simulink model "SSN_39busRT_Ctrl_4WT_19B"  (R2021a)
settings: Solver=ode3  StartTime=0.0  StopTime=10  FixedStep=Ts  MaxStep=1/60  RelTol=1e-2  AbsTol=1e-1
PreLoadFcn:
  | Ts=2.50e-6; ssn_ieee39_params; load('Pwf.mat');
InitFcn:
  | Ts=2.50e-6; ssn_ieee39_params; load('Pwf.mat');
values from neighbouring files (symbols this model uses):
  f = 50    [ssn_ieee39_params_ctrl.m]
  fNom = f    (= 60)    [ssn_ieee39_params_ctrl.m]
  ILR = 5.02    [ssn_ieee39_params_ctrl.m]
  IQMIN = 0.1    [ssn_ieee39_params_ctrl.m]
  ISCLIM = 1    [ssn_ieee39_params_ctrl.m]
  ITFpu = 1.10    (= 1.1)    [ssn_ieee39_params_ctrl.m]
  K = 1    [ssn_ieee39_params_ctrl.m]
  K1 = 1    [ssn_ieee39_params_ctrl.m]
  K2 = 2    [ssn_ieee39_params_ctrl.m]
  KCL = 1.04    [ssn_ieee39_params_ctrl.m]
  KFB = 0    [ssn_ieee39_params_ctrl.m]
  KFF = 1    [ssn_ieee39_params_ctrl.m]
  KFIX = 1    [ssn_ieee39_params_ctrl.m]
  KG = 1    [ssn_ieee39_params_ctrl.m]
  KIA = 59.91    [ssn_ieee39_params_ctrl.m]
  KIOEX = 0.0303    [ssn_ieee39_params_ctrl.m]
  KIUEX = 0.0303    [ssn_ieee39_params_ctrl.m]
  KIUOEX = 1    [ssn_ieee39_params_ctrl.m]
  KIUUEX = 1    [ssn_ieee39_params_ctrl.m]
  KLR = 22.47    [ssn_ieee39_params_ctrl.m]
  KM = 1    [ssn_ieee39_params_ctrl.m]
  KOEL = 0.24    [ssn_ieee39_params_ctrl.m]
  Kp = 1    [ssn_ieee39_params_ctrl.m]
  KPA = 30    [ssn_ieee39_params_ctrl.m]
  KPOEL = 1    [ssn_ieee39_params_ctrl.m]
  KPOEX = 0    [ssn_ieee39_params_ctrl.m]
  KPUEX = 0    [ssn_ieee39_params_ctrl.m]
  KSCALE = 0.319    [ssn_ieee39_params_ctrl.m]
  KUF = 0    [ssn_ieee39_params_ctrl.m]
  KUI = 0.001    [ssn_ieee39_params_ctrl.m]
  KUL = 0.24    [ssn_ieee39_params_ctrl.m]
  s = 10    [ssn_ieee39_params_ctrl.m]
  TA = 0.01    [ssn_ieee39_params_ctrl.m]
  Tadj = 0    [ssn_ieee39_params_ctrl.m]
  taps = [1 1 1.07 1.07 1.009 1.025 1 1.025 1.025 1.025]*1    [ssn_ieee39_params_ctrl.m]
  TF = 0.02    [ssn_ieee39_params_ctrl.m]
  TG = 0.024    [ssn_ieee39_params_ctrl.m]
  TINV = 0    [ssn_ieee39_params_ctrl.m]
  TIT = 0.1    [ssn_ieee39_params_ctrl.m]
  TL_10_11_len = 14    [ssn_ieee39_params_ctrl.m]
  TL_10_13_len = 14    [ssn_ieee39_params_ctrl.m]
  TL_13_14_len = 32    [ssn_ieee39_params_ctrl.m]
  TL_14_15_len = 70    [ssn_ieee39_params_ctrl.m]
  TL_15_16_len = 31.5    [ssn_ieee39_params_ctrl.m]
  TL_16_17_len = 26    [ssn_ieee39_params_ctrl.m]
  TL_16_19_len = 61    [ssn_ieee39_params_ctrl.m]
  TL_16_21_len = 46    [ssn_ieee39_params_ctrl.m]
  TL_16_24_len = 15    [ssn_ieee39_params_ctrl.m]
  TL_17_18_len = 26    [ssn_ieee39_params_ctrl.m]
  TL_17_27_len = 59    [ssn_ieee39_params_ctrl.m]
  TL_1_2_len = 134    [ssn_ieee39_params_ctrl.m]
  TL_1_39_len = 105    [ssn_ieee39_params_ctrl.m]
  TL_21_22_len = 47    [ssn_ieee39_params_ctrl.m]
  TL_22_23_len = 33    [ssn_ieee39_params_ctrl.m]
  TL_24_23_len = 88    [ssn_ieee39_params_ctrl.m]
  TL_25_26_len = 101    [ssn_ieee39_params_ctrl.m]
  TL_26_27_len = 46.5    [ssn_ieee39_params_ctrl.m]
  TL_26_28_len = 151    [ssn_ieee39_params_ctrl.m]
  TL_26_29_len = 200    [ssn_ieee39_params_ctrl.m]
  TL_28_29_len = 48    [ssn_ieee39_params_ctrl.m]
  TL_2_25_len = 28    [ssn_ieee39_params_ctrl.m]
  TL_2_2_len = 49    [ssn_ieee39_params_ctrl.m]
  TL_3_18_len = 42    [ssn_ieee39_params_ctrl.m]
  TL_3_4_len = 53    [ssn_ieee39_params_ctrl.m]
  TL_4_14_len = 33    [ssn_ieee39_params_ctrl.m]
  TL_4_5_len = 32.5    [ssn_ieee39_params_ctrl.m]
  TL_5_6_len = 14    [ssn_ieee39_params_ctrl.m]
  TL_5_8_len = 32    [ssn_ieee39_params_ctrl.m]
  TL_6_11_len = 26.5    [ssn_ieee39_params_ctrl.m]
  TL_6_7_len = 25.5    [ssn_ieee39_params_ctrl.m]
  TL_7_8_len = 15    [ssn_ieee39_params_ctrl.m]
  TL_8_9_len = 93    [ssn_ieee39_params_ctrl.m]
  TL_9_39_len = 136    [ssn_ieee39_params_ctrl.m]
  TOEL = 5.00    (= 5)    [ssn_ieee39_params_ctrl.m]
  TQREF = 0    [ssn_ieee39_params_ctrl.m]
  TQSCL = 0.012    [ssn_ieee39_params_ctrl.m]
  Ts_PMU = 1/1000    (= 0.001)    [ssn_ieee39_params_ctrl.m]
  TU1 = 0    [ssn_ieee39_params_ctrl.m]
  TU2 = 0    [ssn_ieee39_params_ctrl.m]
  TU3 = 0    [ssn_ieee39_params_ctrl.m]
  TU4 = 0    [ssn_ieee39_params_ctrl.m]
  TUL = 0    [ssn_ieee39_params_ctrl.m]
  TUP = 0.050    (= 0.05)    [ssn_ieee39_params_ctrl.m]
  TUQ = .005    (= 0.005)    [ssn_ieee39_params_ctrl.m]
  TUV = 0.2    [ssn_ieee39_params_ctrl.m]
  VAAMAX = VAMAX    (= 7.05)    [ssn_ieee39_params_ctrl.m]
  VAMAX = 7.05    [ssn_ieee39_params_ctrl.m]
  VAMIN = -6.11    [ssn_ieee39_params_ctrl.m]
  VBMAX = 999    [ssn_ieee39_params_ctrl.m]
  VF = 0    [ssn_ieee39_params_ctrl.m]
  VFB = 0    [ssn_ieee39_params_ctrl.m]
  VMMAX = 7.05    [ssn_ieee39_params_ctrl.m]
  VMMIN = -6.11    [ssn_ieee39_params_ctrl.m]
  VOELmax1 = 0.2353    [ssn_ieee39_params_ctrl.m]
  VOELmax2 = 0.0    (= 0)    [ssn_ieee39_params_ctrl.m]
  VOELmin1 = -0.24    [ssn_ieee39_params_ctrl.m]
  VOELmin2 = -1.0    (= -1)    [ssn_ieee39_params_ctrl.m]
  VRMAX = 7.05    [ssn_ieee39_params_ctrl.m]
  VRMIN = -6.11    [ssn_ieee39_params_ctrl.m]
  VSCLmax = 0.20    (= 0.2)    [ssn_ieee39_params_ctrl.m]
  VSCLmin = -0.10    (= -0.1)    [ssn_ieee39_params_ctrl.m]
  VUELmax1 = 1    [ssn_ieee39_params_ctrl.m]
  VUELmax2 = 1    [ssn_ieee39_params_ctrl.m]
  VUELmin1 = -1    [ssn_ieee39_params_ctrl.m]
  VUELmin2 = -1    [ssn_ieee39_params_ctrl.m]
  VUImax = 1    [ssn_ieee39_params_ctrl.m]
  VUImin = -1    [ssn_ieee39_params_ctrl.m]
undefined symbols (not defined in the file or in its folder): another_event_name, D1, Delta, DiscIntNeverNeededParam, find_system, MOV_segment9, my_event_name, powergui, Pw1, Pw2, Pw3, Pw4, vNomHV
libraries: powerlib_extras x162, spsThreePhaseVIMeasurementLib x55, spsCurrentMeasurementLib x52, simulink_extras x44, slpidlib x40, op_dpl_lib x36, spsST2AModel x20, spsThreePhaseParallelRLCLoadLib x20, spsThreePhaseTransformerTwoWindingsLib x17, spsControlledVoltageSourceLib x16, spsVoltageMeasurementLib x12, spsSynchronousMachinepuStandardLib x10
(part 15 of 19)

== system SSN_39busRT_Ctrl_4WT_19B/SM_master/4 WT/SS_windfarm3to4/Wind Farm (DFIG Type)/Wind Turbine Doubly-Fed Induction Generator (Average Model)1/Average_VSC ==
  Uref : Inport
  Converter_model : Subsystem
  Demux : Demux  Outputs=2
  Ia_meas : spsCurrentMeasurementLib/Current Measurement  PhasorSimulation=off  OutputType=Complex  PSBequivalent=0
  Ic_meas : spsCurrentMeasurementLib/Current Measurement  PhasorSimulation=off  OutputType=Complex  PSBequivalent=0
  Idc : spsControlledCurrentSourceLib/Controlled Current Source  Initialize=on  Source_Type=AC  Amplitude=0  Phase=0  Frequency=0  Measurements=None
  Mux : Mux  Inputs=2
  Vab : spsControlledVoltageSourceLib/Controlled Voltage Source  Initialize=on  Source_Type=AC  Amplitude=0  Phase=0  Frequency=0  Measurements=None
  Vbc : spsControlledVoltageSourceLib/Controlled Voltage Source  Initialize=on  Source_Type=AC  Amplitude=0  Phase=0  Frequency=0  Measurements=None
  Vdc_meas : spsVoltageMeasurementLib/Voltage Measurement  PhasorSimulation=off  OutputType=Complex  PSBequivalent=0
  A : PMIOPort  Side=Left
  B : PMIOPort  Port=2  Side=Left
  C : PMIOPort  Port=3  Side=Left
  + : PMIOPort  Port=4  Side=Right
  - : PMIOPort  Port=5  Side=Right
  wires:
  Converter_model/2(Vab_Vbc) -> Demux/1
  Converter_model/1(Idc) -> Idc/1  "Idc"
  Mux/1 -> Converter_model/1(Ia_Ic)
  Vdc_meas/1 -> Converter_model/2(Vdc)
  Uref/1 -> Converter_model/3(Uref)
  Ic_meas/1 -> Mux/2  "Ic"
  Ia_meas/1 -> Mux/1  "Ia"
  Demux/1 -> Vab/1  "Vab"
  Demux/2 -> Vbc/1  "Vbc"
  connections:
  Idc/LConn1 -- -/RConn1 -- Vdc_meas/LConn1
  Idc/RConn1 -- +/RConn1 -- Vdc_meas/LConn2
  C/RConn1 -- Ic_meas/LConn1
  A/RConn1 -- Ia_meas/LConn1
  Ia_meas/RConn1 -- Vab/LConn1
  B/RConn1 -- Vbc/LConn1 -- Vab/RConn1
  Vbc/RConn1 -- Ic_meas/RConn1

== system SSN_39busRT_Ctrl_4WT_19B/SM_master/4 WT/SS_windfarm3to4/Wind Farm (DFIG Type)/Wind Turbine Doubly-Fed Induction Generator (Average Model)1/Average_VSC1 ==
  Uref : Inport
  Converter_model : Subsystem
  Demux : Demux  Outputs=2
  Ia_meas : spsCurrentMeasurementLib/Current Measurement  PhasorSimulation=off  OutputType=Complex  PSBequivalent=0
  Ic_meas : spsCurrentMeasurementLib/Current Measurement  PhasorSimulation=off  OutputType=Complex  PSBequivalent=0
  Idc : spsControlledCurrentSourceLib/Controlled Current Source  Initialize=on  Source_Type=AC  Amplitude=0  Phase=0  Frequency=0  Measurements=None
  Mux : Mux  Inputs=2
  Vab : spsControlledVoltageSourceLib/Controlled Voltage Source  Initialize=on  Source_Type=AC  Amplitude=0  Phase=0  Frequency=0  Measurements=None
  Vbc : spsControlledVoltageSourceLib/Controlled Voltage Source  Initialize=on  Source_Type=AC  Amplitude=0  Phase=0  Frequency=0  Measurements=None
  Vdc_meas : spsVoltageMeasurementLib/Voltage Measurement  PhasorSimulation=off  OutputType=Complex  PSBequivalent=0
  A : PMIOPort  Side=Left
  B : PMIOPort  Port=2  Side=Left
  C : PMIOPort  Port=3  Side=Left
  + : PMIOPort  Port=4  Side=Right
  - : PMIOPort  Port=5  Side=Right
  wires:
  Converter_model/2(Vab_Vbc) -> Demux/1
  Converter_model/1(Idc) -> Idc/1  "Idc"
  Mux/1 -> Converter_model/1(Ia_Ic)
  Vdc_meas/1 -> Converter_model/2(Vdc)
  Uref/1 -> Converter_model/3(Uref)
  Ic_meas/1 -> Mux/2  "Ic"
  Ia_meas/1 -> Mux/1  "Ia"
  Demux/1 -> Vab/1  "Vab"
  Demux/2 -> Vbc/1  "Vbc"
  connections:
  Idc/LConn1 -- -/RConn1 -- Vdc_meas/LConn1
  Idc/RConn1 -- +/RConn1 -- Vdc_meas/LConn2
  C/RConn1 -- Ic_meas/LConn1
  A/RConn1 -- Ia_meas/LConn1
  Ia_meas/RConn1 -- Vab/LConn1
  B/RConn1 -- Vbc/LConn1 -- Vab/RConn1
  Vbc/RConn1 -- Ic_meas/RConn1

== system SSN_39busRT_Ctrl_4WT_19B/SM_master/4 WT/SS_windfarm3to4/Wind Farm (DFIG Type)/Wind Turbine Doubly-Fed Induction Generator (Average Model)1/Control System_average ==
  Vabc_B1 : Inport
  Q_ref : Inport  Port=2
  Iq_grid_conv_ref : Inport  Port=3
  wr : Inport  Port=4
  Iabc_grid_conv : Inport  Port=5
  Iabc_stator : Inport  Port=6
  Iabc_rotor : Inport  Port=7
  Q_B1 : Inport  Port=8
  angle_rotor : Inport  Port=9
  Vdc : Inport  Port=10
  Control : Subsystem
  Filter 1000 Hz : Subsystem  mask{Freq=1000, Zeta=0.707, Ts=Ts}
      mask prompts: Freq "Cut-off frequency (Hz):"; Zeta "Damping factor Zeta:"; Ts "Sample time"
  Unit Delay3 : UnitDelay  SampleTime=Ts  HasFrameUpgradeWarning=on
  Unit Delay4 : UnitDelay  SampleTime=Ts  HasFrameUpgradeWarning=on
  Uref_grid_conv : Outport
  Uref_rotor_conv : Outport  Port=2
  Theta_Freq : Outport  Port=3
  Pitch_angle : Outport  Port=4
  wires:
  wr/1 -> Filter 1000 Hz/9(wr)
  Q_B1/1 -> Filter 1000 Hz/8(Q_B1)
  Iabc_grid_conv/1 -> Filter 1000 Hz/2(Iabc_grid_conv)
  Iabc_rotor/1 -> Filter 1000 Hz/5(Iabc_rotor)
  Filter 1000 Hz/1("Vabc_B1 ") -> Control/1(Vabc_B1)
  Filter 1000 Hz/2("Iabc_grid_conv ") -> Control/2(Iabc_grid_conv)
  Filter 1000 Hz/3("Vdc ") -> Control/3(Vdc)
  Filter 1000 Hz/4("Iabc_stator ") -> Control/4(Iabc_stator)
  Filter 1000 Hz/5("Iabc_rotor ") -> Control/5(Iabc_rotor)
  Filter 1000 Hz/6("Q_ref ") -> Control/6(Q_ref)
  Filter 1000 Hz/7("Iq_grid_conv_ref ") -> Control/7(Iq_grid_conv_ref)
  Filter 1000 Hz/8("Q_B1 ") -> Control/8(Q_B1)
  Filter 1000 Hz/9("wr ") -> Control/9(wr)
  Filter 1000 Hz/10("angle_rotor ") -> Control/10(angle_rotor)
  Vabc_B1/1 -> Filter 1000 Hz/1(Vabc_B1)
  Iabc_stator/1 -> Filter 1000 Hz/4(Iabc_stator)
  Q_ref/1 -> Filter 1000 Hz/6(Q_ref)
  Iq_grid_conv_ref/1 -> Filter 1000 Hz/7(Iq_grid_conv_ref)
  Control/3(Theta_Freq) -> Theta_Freq/1
  Control/4(Pitch_angle) -> Pitch_angle/1
  Control/1(Uctrl_grid_conv) -> Unit Delay4/1
  Control/2(Uctrl_rotor_conv) -> Unit Delay3/1
  Vdc/1 -> Filter 1000 Hz/3(Vdc)
  angle_rotor/1 -> Filter 1000 Hz/10(angle_rotor)
  Unit Delay4/1 -> Uref_grid_conv/1
  Unit Delay3/1 -> Uref_rotor_conv/1

== system SSN_39busRT_Ctrl_4WT_19B/SM_master/4 WT/SS_windfarm3to4/Wind Farm (DFIG Type)/Wind Turbine Doubly-Fed Induction Generator (Average Model)1/Data acquisition electrical ==
  Vabc_B1 : Inport
  Iabc_B1 : Inport  Port=2
  Theta_Freq : Inport  Port=3
  Vdc : Inport  Port=4
  -->pu : Gain  Gain=1/(Pnom*NumberOfUnits)  SaturateOnIntegerOverflow=on  OutDataTypeStr=Inherit: Same as input  ParamDataTypeStr=Inherit: Same as input
  -1 : Gain  Gain=-1  SaturateOnIntegerOverflow=on  OutDataTypeStr=Inherit: Same as input  ParamDataTypeStr=Inherit: Same as input
  Bus Creator : BusCreator  Inputs=5
  Demux1 : Demux  Outputs=2
      settings: DisplayOption=none
  Demux2 : Demux  Outputs=2
      settings: DisplayOption=none
  Discrete 3-phase PLL-Driven Positive-Sequence Active & Reactive Power : powerlib_extras/Discrete Measurements/Discrete 3-phase PLL-Driven  Positive-Sequence Active & Reactive Power  Finit=Fnom  Fmin=45  Par_Vinit=[1 30]  Par_Iinit=[0.5 -10]  Ts=Ts_Control
      settings: SourceProductBaseCode=PS
  Mux : Mux  Inputs=2
  Terminator : Terminator
  Trigonometric Function : Trigonometry
  Trigonometric Function1 : Trigonometry  Operator=cos
  pu->A : Gain  Gain=Pnom*NumberOfUnits/sqrt(3)/Vnom*sqrt(2)  SaturateOnIntegerOverflow=on  OutDataTypeStr=Inherit: Same as input  ParamDataTypeStr=Inherit: Same as input
  pu->V : Gain  Gain=Vnom*sqrt(2)/sqrt(3)  SaturateOnIntegerOverflow=on  OutDataTypeStr=Inherit: Same as input  ParamDataTypeStr=Inherit: Same as input
  meas : Outport
  Q_B1 : Outport  Port=2
  wires:
  Demux2/2 -> Discrete 3-phase PLL-Driven Positive-Sequence Active & Reactive Power/1
  Demux2/1 -> Trigonometric Function1/1, Trigonometric Function/1
  Theta_Freq/1 -> Demux2/1
  Discrete 3-phase PLL-Driven Positive-Sequence Active & Reactive Power/1 -> Terminator/1
  Mux/1 -> Discrete 3-phase PLL-Driven Positive-Sequence Active & Reactive Power/2
  Trigonometric Function1/1 -> Mux/2
  Trigonometric Function/1 -> Mux/1
  pu->V/1 -> Discrete 3-phase PLL-Driven Positive-Sequence Active & Reactive Power/3
  Discrete 3-phase PLL-Driven Positive-Sequence Active & Reactive Power/2 -> -1/1
  pu->A/1 -> Discrete 3-phase PLL-Driven Positive-Sequence Active & Reactive Power/4
  Bus Creator/1 -> meas/1
  Iabc_B1/1 -> pu->A/1, Bus Creator/2  "Iabc_B1"
  Vabc_B1/1 -> pu->V/1, Bus Creator/1  "Vabc_B1"
  Vdc/1 -> Bus Creator/5  "Vdc"
  -1/1 -> Demux1/1
  Demux1/2 -> Bus Creator/4, -->pu/1  "Q_B1"
  Demux1/1 -> Bus Creator/3  "P_B1"
  -->pu/1 -> Q_B1/1

== system SSN_39busRT_Ctrl_4WT_19B/SM_master/4 WT/SS_windfarm3to4/Wind Farm (DFIG Type)/Wind Turbine Doubly-Fed Induction Generator (Average Model)1/Subsystem ==
  Current Measurement : spsCurrentMeasurementLib/Current Measurement  PhasorSimulation=off  OutputType=Complex  PSBequivalent=0
  Current Measurement1 : spsCurrentMeasurementLib/Current Measurement  PhasorSimulation=off  OutputType=Complex  PSBequivalent=0
  Current Measurement2 : spsCurrentMeasurementLib/Current Measurement  PhasorSimulation=off  OutputType=Complex  PSBequivalent=0
  Gain : Gain  Gain=1/(Pnom*NumberOfUnits/(Vnom*sqrt(3)))/sqrt(2)
  Mux : Mux  Inputs=3
  A : PMIOPort  Side=Left
  a : PMIOPort  Port=2  Side=Right
  B : PMIOPort  Port=3  Side=Left
  b : PMIOPort  Port=4  Side=Right
  C : PMIOPort  Port=5  Side=Left
  c : PMIOPort  Port=6  Side=Right
  IabcPU : Outport
  wires:
  Current Measurement2/1 -> Mux/3
  Current Measurement1/1 -> Mux/2
  Current Measurement/1 -> Mux/1
  Mux/1 -> Gain/1
  Gain/1 -> IabcPU/1
  connections:
  A/RConn1 -- Current Measurement/LConn1
  a/RConn1 -- Current Measurement/RConn1
  b/RConn1 -- Current Measurement1/RConn1
  B/RConn1 -- Current Measurement1/LConn1
  C/RConn1 -- Current Measurement2/LConn1
  c/RConn1 -- Current Measurement2/RConn1

== system SSN_39busRT_Ctrl_4WT_19B/SM_master/4 WT/SS_windfarm3to4/Wind Farm (DFIG Type)/Wind Turbine Doubly-Fed Induction Generator (Average Model)1/Subsystem1 ==
  Current Measurement : spsCurrentMeasurementLib/Current Measurement  PhasorSimulation=off  OutputType=Complex  PSBequivalent=0
  Current Measurement1 : spsCurrentMeasurementLib/Current Measurement  PhasorSimulation=off  OutputType=Complex  PSBequivalent=0
  Current Measurement2 : spsCurrentMeasurementLib/Current Measurement  PhasorSimulation=off  OutputType=Complex  PSBequivalent=0
  Gain : Gain  Gain=1/(Pnom*NumberOfUnits/(Vnom*sqrt(3)))/sqrt(2)
  Mux : Mux  Inputs=3
  A : PMIOPort  Side=Left
  a : PMIOPort  Port=2  Side=Right
  B : PMIOPort  Port=3  Side=Left
  b : PMIOPort  Port=4  Side=Right
  C : PMIOPort  Port=5  Side=Left
  c : PMIOPort  Port=6  Side=Right
  IabcPU : Outport
  wires:
  Gain/1 -> IabcPU/1
  Mux/1 -> Gain/1
  Current Measurement/1 -> Mux/1
  Current Measurement1/1 -> Mux/2
  Current Measurement2/1 -> Mux/3
  connections:
  c/RConn1 -- Current Measurement2/RConn1
  C/RConn1 -- Current Measurement2/LConn1
  B/RConn1 -- Current Measurement1/LConn1
  b/RConn1 -- Current Measurement1/RConn1
  a/RConn1 -- Current Measurement/RConn1
  A/RConn1 -- Current Measurement/LConn1

== system SSN_39busRT_Ctrl_4WT_19B/SM_master/4 WT/SS_windfarm3to4/Wind Farm (DFIG Type)/Wind Turbine Doubly-Fed Induction Generator (Average Model)1/Subsystem2 ==
  Current Measurement : spsCurrentMeasurementLib/Current Measurement  PhasorSimulation=off  OutputType=Complex  PSBequivalent=0
  Current Measurement1 : spsCurrentMeasurementLib/Current Measurement  PhasorSimulation=off  OutputType=Complex  PSBequivalent=0
  Current Measurement2 : spsCurrentMeasurementLib/Current Measurement  PhasorSimulation=off  OutputType=Complex  PSBequivalent=0
  Gain : Gain  Gain=1/(Pnom*NumberOfUnits/(Vnom*sqrt(3)))/sqrt(2)
  Mux : Mux  Inputs=3
  A : PMIOPort  Side=Left
  a : PMIOPort  Port=2  Side=Right
  B : PMIOPort  Port=3  Side=Left
  b : PMIOPort  Port=4  Side=Right
  C : PMIOPort  Port=5  Side=Left
  c : PMIOPort  Port=6  Side=Right
  IabcPU : Outport
  wires:
  Current Measurement2/1 -> Mux/3
  Current Measurement1/1 -> Mux/2
  Current Measurement/1 -> Mux/1
  Mux/1 -> Gain/1
  Gain/1 -> IabcPU/1
  connections:
  A/RConn1 -- Current Measurement/LConn1
  a/RConn1 -- Current Measurement/RConn1
  b/RConn1 -- Current Measurement1/RConn1
  B/RConn1 -- Current Measurement1/LConn1
  C/RConn1 -- Current Measurement2/LConn1
  c/RConn1 -- Current Measurement2/RConn1

== system SSN_39busRT_Ctrl_4WT_19B/SM_master/4 WT/SS_windfarm3to4/Wind Farm (DFIG Type)/Wind Turbine Doubly-Fed Induction Generator (Average Model)1/Wind Turbine v ==
  Generator speed (pu) : Inport
  Wind Power : Inport  Port=2
  Avoid division by zero : Saturate  UpperLimit=1e6  LowerLimit=1e-6
  Gain : Gain  Gain=-1  SaturateOnIntegerOverflow=on  OutDataTypeStr=Inherit: Same as input  ParamDataTypeStr=Inherit: Same as input
  Product2 : Product  Inputs=*/  InputSameDT=on  SaturateOnIntegerOverflow=on  OutDataTypeStr=Inherit: Same as first input
  pu->pu : Gain  Gain=P_wind_base*Pnom/Pelec_base  SaturateOnIntegerOverflow=on  OutDataTypeStr=Inherit: Same as input  ParamDataTypeStr=Inherit: Same as input
  Tm (pu) : Outport
  wires:
  Generator speed (pu)/1 -> Avoid division by zero/1
  pu->pu/1 -> Product2/1
  Gain/1 -> Tm (pu)/1
  Avoid division by zero/1 -> Product2/2
  Product2/1 -> Gain/1
  Wind Power/1 -> pu->pu/1

== system SSN_39busRT_Ctrl_4WT_19B/SM_master/4 WT/SS_windfarm3to4/Wind Farm (DFIG Type)2/Wind Turbine Doubly-Fed Induction Generator (Average Model)1/Average_VSC ==
  Uref : Inport
  Converter_model : Subsystem
  Demux : Demux  Outputs=2
  Ia_meas : spsCurrentMeasurementLib/Current Measurement  PhasorSimulation=off  OutputType=Complex  PSBequivalent=0
  Ic_meas : spsCurrentMeasurementLib/Current Measurement  PhasorSimulation=off  OutputType=Complex  PSBequivalent=0
  Idc : spsControlledCurrentSourceLib/Controlled Current Source  Initialize=on  Source_Type=AC  Amplitude=0  Phase=0  Frequency=0  Measurements=None
  Mux : Mux  Inputs=2
  Vab : spsControlledVoltageSourceLib/Controlled Voltage Source  Initialize=on  Source_Type=AC  Amplitude=0  Phase=0  Frequency=0  Measurements=None
  Vbc : spsControlledVoltageSourceLib/Controlled Voltage Source  Initialize=on  Source_Type=AC  Amplitude=0  Phase=0  Frequency=0  Measurements=None
  Vdc_meas : spsVoltageMeasurementLib/Voltage Measurement  PhasorSimulation=off  OutputType=Complex  PSBequivalent=0
  A : PMIOPort  Side=Left
  B : PMIOPort  Port=2  Side=Left
  C : PMIOPort  Port=3  Side=Left
  + : PMIOPort  Port=4  Side=Right
  - : PMIOPort  Port=5  Side=Right
  wires:
  Demux/2 -> Vbc/1  "Vbc"
  Demux/1 -> Vab/1  "Vab"
  Ia_meas/1 -> Mux/1  "Ia"
  Ic_meas/1 -> Mux/2  "Ic"
  Uref/1 -> Converter_model/3(Uref)
  Vdc_meas/1 -> Converter_model/2(Vdc)
  Mux/1 -> Converter_model/1(Ia_Ic)
  Converter_model/1(Idc) -> Idc/1  "Idc"
  Converter_model/2(Vab_Vbc) -> Demux/1
  connections:
  Vbc/RConn1 -- Ic_meas/RConn1
  Vab/RConn1 -- Vbc/LConn1 -- B/RConn1
  Ia_meas/RConn1 -- Vab/LConn1
  A/RConn1 -- Ia_meas/LConn1
  C/RConn1 -- Ic_meas/LConn1
  Vdc_meas/LConn2 -- +/RConn1 -- Idc/RConn1
  Vdc_meas/LConn1 -- -/RConn1 -- Idc/LConn1

== system SSN_39busRT_Ctrl_4WT_19B/SM_master/4 WT/SS_windfarm3to4/Wind Farm (DFIG Type)2/Wind Turbine Doubly-Fed Induction Generator (Average Model)1/Average_VSC1 ==
  Uref : Inport
  Converter_model : Subsystem
  Demux : Demux  Outputs=2
  Ia_meas : spsCurrentMeasurementLib/Current Measurement  PhasorSimulation=off  OutputType=Complex  PSBequivalent=0
  Ic_meas : spsCurrentMeasurementLib/Current Measurement  PhasorSimulation=off  OutputType=Complex  PSBequivalent=0
  Idc : spsControlledCurrentSourceLib/Controlled Current Source  Initialize=on  Source_Type=AC  Amplitude=0  Phase=0  Frequency=0  Measurements=None
  Mux : Mux  Inputs=2
  Vab : spsControlledVoltageSourceLib/Controlled Voltage Source  Initialize=on  Source_Type=AC  Amplitude=0  Phase=0  Frequency=0  Measurements=None
  Vbc : spsControlledVoltageSourceLib/Controlled Voltage Source  Initialize=on  Source_Type=AC  Amplitude=0  Phase=0  Frequency=0  Measurements=None
  Vdc_meas : spsVoltageMeasurementLib/Voltage Measurement  PhasorSimulation=off  OutputType=Complex  PSBequivalent=0
  A : PMIOPort  Side=Left
  B : PMIOPort  Port=2  Side=Left
  C : PMIOPort  Port=3  Side=Left
  + : PMIOPort  Port=4  Side=Right
  - : PMIOPort  Port=5  Side=Right
  wires:
  Demux/2 -> Vbc/1  "Vbc"
  Demux/1 -> Vab/1  "Vab"
  Ia_meas/1 -> Mux/1  "Ia"
  Ic_meas/1 -> Mux/2  "Ic"
  Uref/1 -> Converter_model/3(Uref)
  Vdc_meas/1 -> Converter_model/2(Vdc)
  Mux/1 -> Converter_model/1(Ia_Ic)
  Converter_model/1(Idc) -> Idc/1  "Idc"
  Converter_model/2(Vab_Vbc) -> Demux/1
  connections:
  Vbc/RConn1 -- Ic_meas/RConn1
  Vab/RConn1 -- Vbc/LConn1 -- B/RConn1
  Ia_meas/RConn1 -- Vab/LConn1
  A/RConn1 -- Ia_meas/LConn1
  C/RConn1 -- Ic_meas/LConn1
  Vdc_meas/LConn2 -- +/RConn1 -- Idc/RConn1
  Vdc_meas/LConn1 -- -/RConn1 -- Idc/LConn1

== system SSN_39busRT_Ctrl_4WT_19B/SM_master/4 WT/SS_windfarm3to4/Wind Farm (DFIG Type)2/Wind Turbine Doubly-Fed Induction Generator (Average Model)1/Control System_average ==
  Vabc_B1 : Inport
  Q_ref : Inport  Port=2
  Iq_grid_conv_ref : Inport  Port=3
  wr : Inport  Port=4
  Iabc_grid_conv : Inport  Port=5
  Iabc_stator : Inport  Port=6
  Iabc_rotor : Inport  Port=7
  Q_B1 : Inport  Port=8
  angle_rotor : Inport  Port=9
  Vdc : Inport  Port=10
  Control : Subsystem
  Filter 1000 Hz : Subsystem  mask{Freq=1000, Zeta=0.707, Ts=Ts}
      mask prompts: Freq "Cut-off frequency (Hz):"; Zeta "Damping factor Zeta:"; Ts "Sample time"
  Unit Delay3 : UnitDelay  SampleTime=Ts  HasFrameUpgradeWarning=on
  Unit Delay4 : UnitDelay  SampleTime=Ts  HasFrameUpgradeWarning=on
  Uref_grid_conv : Outport
  Uref_rotor_conv : Outport  Port=2
  Theta_Freq : Outport  Port=3
  Pitch_angle : Outport  Port=4
  wires:
  Unit Delay3/1 -> Uref_rotor_conv/1
  Unit Delay4/1 -> Uref_grid_conv/1
  angle_rotor/1 -> Filter 1000 Hz/10(angle_rotor)
  Vdc/1 -> Filter 1000 Hz/3(Vdc)
  Control/2(Uctrl_rotor_conv) -> Unit Delay3/1
  Control/1(Uctrl_grid_conv) -> Unit Delay4/1
  Control/4(Pitch_angle) -> Pitch_angle/1
  Control/3(Theta_Freq) -> Theta_Freq/1
  Iq_grid_conv_ref/1 -> Filter 1000 Hz/7(Iq_grid_conv_ref)
  Q_ref/1 -> Filter 1000 Hz/6(Q_ref)
  Iabc_stator/1 -> Filter 1000 Hz/4(Iabc_stator)
  Vabc_B1/1 -> Filter 1000 Hz/1(Vabc_B1)
  Filter 1000 Hz/10("angle_rotor ") -> Control/10(angle_rotor)
  Filter 1000 Hz/9("wr ") -> Control/9(wr)
  Filter 1000 Hz/8("Q_B1 ") -> Control/8(Q_B1)
  Filter 1000 Hz/7("Iq_grid_conv_ref ") -> Control/7(Iq_grid_conv_ref)
  Filter 1000 Hz/6("Q_ref ") -> Control/6(Q_ref)
  Filter 1000 Hz/5("Iabc_rotor ") -> Control/5(Iabc_rotor)
  Filter 1000 Hz/4("Iabc_stator ") -> Control/4(Iabc_stator)
  Filter 1000 Hz/3("Vdc ") -> Control/3(Vdc)
  Filter 1000 Hz/2("Iabc_grid_conv ") -> Control/2(Iabc_grid_conv)
  Filter 1000 Hz/1("Vabc_B1 ") -> Control/1(Vabc_B1)
  Iabc_rotor/1 -> Filter 1000 Hz/5(Iabc_rotor)
  Iabc_grid_conv/1 -> Filter 1000 Hz/2(Iabc_grid_conv)
  Q_B1/1 -> Filter 1000 Hz/8(Q_B1)
  wr/1 -> Filter 1000 Hz/9(wr)

== system SSN_39busRT_Ctrl_4WT_19B/SM_master/4 WT/SS_windfarm3to4/Wind Farm (DFIG Type)2/Wind Turbine Doubly-Fed Induction Generator (Average Model)1/Data acquisition electrical ==
  Vabc_B1 : Inport
  Iabc_B1 : Inport  Port=2
  Theta_Freq : Inport  Port=3
  Vdc : Inport  Port=4
  -->pu : Gain  Gain=1/(Pnom*NumberOfUnits)  SaturateOnIntegerOverflow=on  OutDataTypeStr=Inherit: Same as input  ParamDataTypeStr=Inherit: Same as input
  -1 : Gain  Gain=-1  SaturateOnIntegerOverflow=on  OutDataTypeStr=Inherit: Same as input  ParamDataTypeStr=Inherit: Same as input
  Bus Creator : BusCreator  Inputs=5
  Demux1 : Demux  Outputs=2
      settings: DisplayOption=none
  Demux2 : Demux  Outputs=2
      settings: DisplayOption=none
  Discrete 3-phase PLL-Driven Positive-Sequence Active & Reactive Power : powerlib_extras/Discrete Measurements/Discrete 3-phase PLL-Driven  Positive-Sequence Active & Reactive Power  Finit=Fnom  Fmin=45  Par_Vinit=[1 30]  Par_Iinit=[0.5 -10]  Ts=Ts_Control
      settings: SourceProductBaseCode=PS
  Mux : Mux  Inputs=2
  Terminator : Terminator
  Trigonometric Function : Trigonometry
  Trigonometric Function1 : Trigonometry  Operator=cos
  pu->A : Gain  Gain=Pnom*NumberOfUnits/sqrt(3)/Vnom*sqrt(2)  SaturateOnIntegerOverflow=on  OutDataTypeStr=Inherit: Same as input  ParamDataTypeStr=Inherit: Same as input
  pu->V : Gain  Gain=Vnom*sqrt(2)/sqrt(3)  SaturateOnIntegerOverflow=on  OutDataTypeStr=Inherit: Same as input  ParamDataTypeStr=Inherit: Same as input
  meas : Outport
  Q_B1 : Outport  Port=2
  wires:
  -->pu/1 -> Q_B1/1
  Demux1/1 -> Bus Creator/3  "P_B1"
  Demux1/2 -> -->pu/1, Bus Creator/4  "Q_B1"
  -1/1 -> Demux1/1
  Vdc/1 -> Bus Creator/5  "Vdc"
  Vabc_B1/1 -> Bus Creator/1, pu->V/1  "Vabc_B1"
  Iabc_B1/1 -> Bus Creator/2, pu->A/1  "Iabc_B1"
  Bus Creator/1 -> meas/1
  pu->A/1 -> Discrete 3-phase PLL-Driven Positive-Sequence Active & Reactive Power/4
  Discrete 3-phase PLL-Driven Positive-Sequence Active & Reactive Power/2 -> -1/1
  pu->V/1 -> Discrete 3-phase PLL-Driven Positive-Sequence Active & Reactive Power/3
  Trigonometric Function/1 -> Mux/1
  Trigonometric Function1/1 -> Mux/2
  Mux/1 -> Discrete 3-phase PLL-Driven Positive-Sequence Active & Reactive Power/2
  Discrete 3-phase PLL-Driven Positive-Sequence Active & Reactive Power/1 -> Terminator/1
  Theta_Freq/1 -> Demux2/1
  Demux2/1 -> Trigonometric Function/1, Trigonometric Function1/1
  Demux2/2 -> Discrete 3-phase PLL-Driven Positive-Sequence Active & Reactive Power/1

== system SSN_39busRT_Ctrl_4WT_19B/SM_master/4 WT/SS_windfarm3to4/Wind Farm (DFIG Type)2/Wind Turbine Doubly-Fed Induction Generator (Average Model)1/Subsystem ==
  Current Measurement : spsCurrentMeasurementLib/Current Measurement  PhasorSimulation=off  OutputType=Complex  PSBequivalent=0
  Current Measurement1 : spsCurrentMeasurementLib/Current Measurement  PhasorSimulation=off  OutputType=Complex  PSBequivalent=0
  Current Measurement2 : spsCurrentMeasurementLib/Current Measurement  PhasorSimulation=off  OutputType=Complex  PSBequivalent=0
  Gain : Gain  Gain=1/(Pnom*NumberOfUnits/(Vnom*sqrt(3)))/sqrt(2)
  Mux : Mux  Inputs=3
  A : PMIOPort  Side=Left
  a : PMIOPort  Port=2  Side=Right
  B : PMIOPort  Port=3  Side=Left
  b : PMIOPort  Port=4  Side=Right
  C : PMIOPort  Port=5  Side=Left
  c : PMIOPort  Port=6  Side=Right
  IabcPU : Outport
  wires:
  Gain/1 -> IabcPU/1
  Mux/1 -> Gain/1
  Current Measurement/1 -> Mux/1
  Current Measurement1/1 -> Mux/2
  Current Measurement2/1 -> Mux/3
  connections:
  c/RConn1 -- Current Measurement2/RConn1
  C/RConn1 -- Current Measurement2/LConn1
  B/RConn1 -- Current Measurement1/LConn1
  b/RConn1 -- Current Measurement1/RConn1
  a/RConn1 -- Current Measurement/RConn1
  A/RConn1 -- Current Measurement/LConn1

== system SSN_39busRT_Ctrl_4WT_19B/SM_master/4 WT/SS_windfarm3to4/Wind Farm (DFIG Type)2/Wind Turbine Doubly-Fed Induction Generator (Average Model)1/Subsystem1 ==
  Current Measurement : spsCurrentMeasurementLib/Current Measurement  PhasorSimulation=off  OutputType=Complex  PSBequivalent=0
  Current Measurement1 : spsCurrentMeasurementLib/Current Measurement  PhasorSimulation=off  OutputType=Complex  PSBequivalent=0
  Current Measurement2 : spsCurrentMeasurementLib/Current Measurement  PhasorSimulation=off  OutputType=Complex  PSBequivalent=0
  Gain : Gain  Gain=1/(Pnom*NumberOfUnits/(Vnom*sqrt(3)))/sqrt(2)
  Mux : Mux  Inputs=3
  A : PMIOPort  Side=Left
  a : PMIOPort  Port=2  Side=Right
  B : PMIOPort  Port=3  Side=Left
  b : PMIOPort  Port=4  Side=Right
  C : PMIOPort  Port=5  Side=Left
  c : PMIOPort  Port=6  Side=Right
  IabcPU : Outport
  wires:
  Current Measurement2/1 -> Mux/3
  Current Measurement1/1 -> Mux/2
  Current Measurement/1 -> Mux/1
  Mux/1 -> Gain/1
  Gain/1 -> IabcPU/1
  connections:
  A/RConn1 -- Current Measurement/LConn1
  a/RConn1 -- Current Measurement/RConn1
  b/RConn1 -- Current Measurement1/RConn1
  B/RConn1 -- Current Measurement1/LConn1
  C/RConn1 -- Current Measurement2/LConn1
  c/RConn1 -- Current Measurement2/RConn1

== system SSN_39busRT_Ctrl_4WT_19B/SM_master/4 WT/SS_windfarm3to4/Wind Farm (DFIG Type)2/Wind Turbine Doubly-Fed Induction Generator (Average Model)1/Subsystem2 ==
  Current Measurement : spsCurrentMeasurementLib/Current Measurement  PhasorSimulation=off  OutputType=Complex  PSBequivalent=0
  Current Measurement1 : spsCurrentMeasurementLib/Current Measurement  PhasorSimulation=off  OutputType=Complex  PSBequivalent=0
  Current Measurement2 : spsCurrentMeasurementLib/Current Measurement  PhasorSimulation=off  OutputType=Complex  PSBequivalent=0
  Gain : Gain  Gain=1/(Pnom*NumberOfUnits/(Vnom*sqrt(3)))/sqrt(2)
  Mux : Mux  Inputs=3
  A : PMIOPort  Side=Left
  a : PMIOPort  Port=2  Side=Right
  B : PMIOPort  Port=3  Side=Left
  b : PMIOPort  Port=4  Side=Right
  C : PMIOPort  Port=5  Side=Left
  c : PMIOPort  Port=6  Side=Right
  IabcPU : Outport
  wires:
  Gain/1 -> IabcPU/1
  Mux/1 -> Gain/1
  Current Measurement/1 -> Mux/1
  Current Measurement1/1 -> Mux/2
  Current Measurement2/1 -> Mux/3
  connections:
  c/RConn1 -- Current Measurement2/RConn1
  C/RConn1 -- Current Measurement2/LConn1
  B/RConn1 -- Current Measurement1/LConn1
  b/RConn1 -- Current Measurement1/RConn1
  a/RConn1 -- Current Measurement/RConn1
  A/RConn1 -- Current Measurement/LConn1

== system SSN_39busRT_Ctrl_4WT_19B/SM_master/4 WT/SS_windfarm3to4/Wind Farm (DFIG Type)2/Wind Turbine Doubly-Fed Induction Generator (Average Model)1/Wind Turbine v ==
  Generator speed (pu) : Inport
  Wind Power : Inport  Port=2
  Avoid division by zero : Saturate  UpperLimit=1e6  LowerLimit=1e-6
  Gain : Gain  Gain=-1  SaturateOnIntegerOverflow=on  OutDataTypeStr=Inherit: Same as input  ParamDataTypeStr=Inherit: Same as input
  Product2 : Product  Inputs=*/  InputSameDT=on  SaturateOnIntegerOverflow=on  OutDataTypeStr=Inherit: Same as first input
  pu->pu : Gain  Gain=P_wind_base*Pnom/Pelec_base  SaturateOnIntegerOverflow=on  OutDataTypeStr=Inherit: Same as input  ParamDataTypeStr=Inherit: Same as input
  Tm (pu) : Outport
  wires:
  Product2/1 -> Gain/1
  Avoid division by zero/1 -> Product2/2
  Gain/1 -> Tm (pu)/1
  pu->pu/1 -> Product2/1
  Generator speed (pu)/1 -> Avoid division by zero/1
  Wind Power/1 -> pu->pu/1

== system SSN_39busRT_Ctrl_4WT_19B/SM_master/4 WT/SS_windfarm1to2/Wind Farm (DFIG Type)/Wind Turbine Doubly-Fed Induction Generator (Average Model)1/Average_VSC/Converter_model ==
  note: P = Vab*Ia -Vbc*Ic = Vdc*Idc
      | Idc = (Vab*Ia -Vbc*Ic)/Vdc
  Ia_Ic : Inport
  Vdc : Inport  Port=2
  Uref : Inport  Port=3
  Add : Sum  Inputs=+-
  Add1 : Sum  Inputs=+-
  Constant : Constant  Value=1e-6
  Delay1 : UnitDelay  SampleTime=Ts  HasFrameUpgradeWarning=on
  Delay2 : UnitDelay  InitialCondition=1e-6  SampleTime=Ts  HasFrameUpgradeWarning=on
  Demux : Demux  Outputs=3
  Demux1 : Demux  Outputs=2
  Gain : Gain  Gain=0.5
  Mult : Product  Inputs=**
  Mux1 : Mux  Inputs=2
  Predictor : Subsystem
  Product3 : Product  RndMeth=Zero
  Product4 : Product  RndMeth=Zero
  Product5 : Product  Inputs=*/  RndMeth=Zero
  Subtract2 : Sum  Inputs=+-
  Subtract3 : Sum
  Idc : Outport
  Vab_Vbc : Outport  Port=2
  wires:
  Delay1/1 -> Gain/1, Predictor/1(In)
  Gain/1 -> Mult/2
  Mult/1 -> Demux/1
  Demux/3 -> Add1/2
  Demux/2 -> Add/2, Add1/1
  Demux/1 -> Add/1
  Predictor/1(Out) -> Subtract3/1
  Add/1 -> Mux1/1, Product3/1  "Vab"
  Add1/1 -> Mux1/2, Product4/1  "Vbc"
  Demux1/2 -> Product4/2  "ic"
  Product3/1 -> Subtract2/1
  Product4/1 -> Subtract2/2
  Subtract3/1 -> Product5/2
  Constant/1 -> Subtract3/2
  Product5/1 -> Delay2/1
  Subtract2/1 -> Product5/1  "Pac"
  Demux1/1 -> Product3/2  "ia"
  Delay2/1 -> Idc/1  "idc"
  Ia_Ic/1 -> Demux1/1
  Vdc/1 -> Delay1/1
  Uref/1 -> Mult/1
  Mux1/1 -> Vab_Vbc/1

== system SSN_39busRT_Ctrl_4WT_19B/SM_master/4 WT/SS_windfarm1to2/Wind Farm (DFIG Type)/Wind Turbine Doubly-Fed Induction Generator (Average Model)1/Average_VSC1/Converter_model ==
  note: P = Vab*Ia -Vbc*Ic = Vdc*Idc
      | Idc = (Vab*Ia -Vbc*Ic)/Vdc
  Ia_Ic : Inport
  Vdc : Inport  Port=2
  Uref : Inport  Port=3
  Add : Sum  Inputs=+-
  Add1 : Sum  Inputs=+-
  Constant : Constant  Value=1e-6
  Delay1 : UnitDelay  SampleTime=Ts  HasFrameUpgradeWarning=on
  Delay2 : UnitDelay  InitialCondition=1e-6  SampleTime=Ts  HasFrameUpgradeWarning=on
  Demux : Demux  Outputs=3
  Demux1 : Demux  Outputs=2
  Gain : Gain  Gain=0.5
  Mult : Product  Inputs=**
  Mux1 : Mux  Inputs=2
  Predictor : Subsystem
  Product3 : Product  RndMeth=Zero
  Product4 : Product  RndMeth=Zero
  Product5 : Product  Inputs=*/  RndMeth=Zero
  Subtract2 : Sum  Inputs=+-
  Subtract3 : Sum
  Idc : Outport
  Vab_Vbc : Outport  Port=2
  wires:
  Delay1/1 -> Gain/1, Predictor/1(In)
  Gain/1 -> Mult/2
  Mult/1 -> Demux/1
  Demux/3 -> Add1/2
  Demux/2 -> Add/2, Add1/1
  Demux/1 -> Add/1
  Predictor/1(Out) -> Subtract3/1
  Add/1 -> Mux1/1, Product3/1  "Vab"
  Add1/1 -> Mux1/2, Product4/1  "Vbc"
  Demux1/2 -> Product4/2  "ic"
  Product3/1 -> Subtract2/1
  Product4/1 -> Subtract2/2
  Subtract3/1 -> Product5/2
  Constant/1 -> Subtract3/2
  Product5/1 -> Delay2/1
  Subtract2/1 -> Product5/1  "Pac"
  Demux1/1 -> Product3/2  "ia"
  Delay2/1 -> Idc/1  "idc"
  Ia_Ic/1 -> Demux1/1
  Vdc/1 -> Delay1/1
  Uref/1 -> Mult/1
  Mux1/1 -> Vab_Vbc/1

== system SSN_39busRT_Ctrl_4WT_19B/SM_master/4 WT/SS_windfarm1to2/Wind Farm (DFIG Type)/Wind Turbine Doubly-Fed Induction Generator (Average Model)1/Control System_average/Control ==
  Vabc_B1 : Inport
  Iabc_grid_conv : Inport  Port=2
  Vdc : Inport  Port=3
  Iabc_stator : Inport  Port=4
  Iabc_rotor : Inport  Port=5
  Q_ref : Inport  Port=6
  Iq_grid_conv_ref : Inport  Port=7
  Q_B1 : Inport  Port=8
  wr : Inport  Port=9
  angle_rotor : Inport  Port=10
  0-pitch_max : Saturate  UpperLimit=pitch_max  LowerLimit=0
  Constant2 : Constant  Value=speed_D
  Discrete 3-phase PLL : powerlib_extras/Discrete  Control Blocks/Discrete 3-phase PLL  Fmin=Fnom-10  Par_Init=[-45 Fnom]  ParK=[60 1400]  Ts=Ts  AGC=off
      settings: SourceProductBaseCode=PS
  Grid-side converter Control system : Subsystem
  Mux : Mux  Inputs=2
  "Rate Limiter   " : RateLimiter  RisingSlewLimit=pitch_rate  FallingSlewLimit=-pitch_rate
  Rotor-side converter Control system : Subsystem
  Sum : Sum  Inputs=|+-  SaturateOnIntegerOverflow=on
  Terminator : Terminator
  pitch_gain : Gain  Gain=pitch_gain  SaturateOnIntegerOverflow=on  OutDataTypeStr=Inherit: Same as input  ParamDataTypeStr=Inherit: Same as input
  Uctrl_grid_conv : Outport
  Uctrl_rotor_conv : Outport  Port=2
  Theta_Freq : Outport  Port=3
  Pitch_angle : Outport  Port=4
  wires:
  Vdc/1 -> Grid-side converter Control system/4(Vdc), Rotor-side converter Control system/2(Vdc)
  Vabc_B1/1 -> Grid-side converter Control system/1(Vabc_B1), Discrete 3-phase PLL/1
  Iq_grid_conv_ref/1 -> Grid-side converter Control system/5(Iq_ref)
  Iabc_grid_conv/1 -> Grid-side converter Control system/2(Iabc_grid_conv), Rotor-side converter Control system/6(Iabc_grid_conv)
  Iabc_stator/1 -> Rotor-side converter Control system/4(Iabc_stator)
  Iabc_rotor/1 -> Rotor-side converter Control system/5(Iabc_rotor)
  Q_ref/1 -> Rotor-side converter Control system/7(Q_ref)
  Discrete 3-phase PLL/2 -> Grid-side converter Control system/3(Theta), Mux/1, Rotor-side converter Control system/3(Theta)
  Mux/1 -> Theta_Freq/1
  Discrete 3-phase PLL/3 -> Terminator/1
  Discrete 3-phase PLL/1 -> Grid-side converter Control system/6(Freq), Mux/2, Rotor-side converter Control system/10(Freq)
  "Rate Limiter   "/1 -> Pitch_angle/1
  pitch_gain/1 -> 0-pitch_max/1
  Sum/1 -> pitch_gain/1
  Constant2/1 -> Sum/2
  0-pitch_max/1 -> "Rate Limiter   "/1
  wr/1 -> Sum/1, Rotor-side converter Control system/1(wr)
  Q_B1/1 -> Rotor-side converter Control system/8(Q_B1)
  angle_rotor/1 -> Rotor-side converter Control system/9(angle_rotor)
  Grid-side converter Control system/2(Vdqs) -> [Vdqs]
  [Vdqs] -> Rotor-side converter Control system/11(Vdqs)
  Grid-side converter Control system/1(Uctrl_grid_conv) -> Uctrl_grid_conv/1
  Rotor-side converter Control system/1(Uctrl_rotor_conv) -> Uctrl_rotor_conv/1

== system SSN_39busRT_Ctrl_4WT_19B/SM_master/4 WT/SS_windfarm1to2/Wind Farm (DFIG Type)/Wind Turbine Doubly-Fed Induction Generator (Average Model)1/Control System_average/Filter 1000 Hz ==
  Vabc_B1 : Inport
  Iabc_grid_conv : Inport  Port=2
  Vdc : Inport  Port=3
  Iabc_stator : Inport  Port=4
  Iabc_rotor : Inport  Port=5
  Q_ref : Inport  Port=6
  Iq_grid_conv_ref : Inport  Port=7
  Q_B1 : Inport  Port=8
  wr : Inport  Port=9
  angle_rotor : Inport  Port=10
  Demux{,1..3} (4 alike) : Demux  Outputs=3
      settings: DisplayOption=none
  Discrete 2nd-Order Filter{1..14,16..18,20} (18 alike) : powerlib_extras/Discrete  Control Blocks/Discrete  2nd-Order Filter  FilterType=Lowpass  Fo=Freq  Zeta=Zeta  Ts=Ts  Initialize=off  Vac_Init=[0.8 -25 60]  Vdc_Init=-0.4  PlotResponse=off  param1=[1 500 1]
      settings: SourceProductBaseCode=PS
  Mux{,1..3} (4 alike) : Mux  Inputs=3
  "Vabc_B1 " : Outport
  "Iabc_grid_conv " : Outport  Port=2
  "Vdc " : Outport  Port=3
  "Iabc_stator " : Outport  Port=4
  "Iabc_rotor " : Outport  Port=5
  "Q_ref " : Outport  Port=6
  "Iq_grid_conv_ref " : Outport  Port=7
  "Q_B1 " : Outport  Port=8
  "wr " : Outport  Port=9
  "angle_rotor " : Outport  Port=10
  wires:
  Demux/1 -> Discrete 2nd-Order Filter1/1
  Demux/2 -> Discrete 2nd-Order Filter2/1
  Demux/3 -> Discrete 2nd-Order Filter3/1
  Discrete 2nd-Order Filter1/1 -> Mux/1
  Discrete 2nd-Order Filter2/1 -> Mux/2
  Discrete 2nd-Order Filter3/1 -> Mux/3
  Vabc_B1/1 -> Demux/1
  Mux/1 -> "Vabc_B1 "/1
  Demux1/1 -> Discrete 2nd-Order Filter4/1
  Demux1/2 -> Discrete 2nd-Order Filter5/1
  Demux1/3 -> Discrete 2nd-Order Filter6/1
  Discrete 2nd-Order Filter4/1 -> Mux1/1
  Discrete 2nd-Order Filter5/1 -> Mux1/2
  Discrete 2nd-Order Filter6/1 -> Mux1/3
  Iabc_grid_conv/1 -> Demux1/1
  Mux1/1 -> "Iabc_grid_conv "/1
  Vdc/1 -> Discrete 2nd-Order Filter7/1
  Discrete 2nd-Order Filter7/1 -> "Vdc "/1
  Demux2/1 -> Discrete 2nd-Order Filter8/1
  Demux2/2 -> Discrete 2nd-Order Filter9/1
  Demux2/3 -> Discrete 2nd-Order Filter10/1
  Discrete 2nd-Order Filter8/1 -> Mux2/1
  Discrete 2nd-Order Filter9/1 -> Mux2/2
  Discrete 2nd-Order Filter10/1 -> Mux2/3
  Iabc_stator/1 -> Demux2/1
  Mux2/1 -> "Iabc_stator "/1
  Q_ref/1 -> Discrete 2nd-Order Filter11/1
  Q_B1/1 -> Discrete 2nd-Order Filter12/1
  Discrete 2nd-Order Filter12/1 -> "Q_B1 "/1
  wr/1 -> Discrete 2nd-Order Filter13/1
  Discrete 2nd-Order Filter13/1 -> "wr "/1
  angle_rotor/1 -> Discrete 2nd-Order Filter14/1
  Discrete 2nd-Order Filter14/1 -> "angle_rotor "/1
  Discrete 2nd-Order Filter11/1 -> "Q_ref "/1
  Demux3/1 -> Discrete 2nd-Order Filter17/1
  Demux3/2 -> Discrete 2nd-Order Filter18/1
  Demux3/3 -> Discrete 2nd-Order Filter16/1
  Discrete 2nd-Order Filter17/1 -> Mux3/1
  Discrete 2nd-Order Filter18/1 -> Mux3/2
  Discrete 2nd-Order Filter16/1 -> Mux3/3
  Iabc_rotor/1 -> Demux3/1
  Mux3/1 -> "Iabc_rotor "/1
  Iq_grid_conv_ref/1 -> Discrete 2nd-Order Filter20/1
  Discrete 2nd-Order Filter20/1 -> "Iq_grid_conv_ref "/1

== system SSN_39busRT_Ctrl_4WT_19B/SM_master/4 WT/SS_windfarm1to2/Wind Farm (DFIG Type)1/Wind Turbine Doubly-Fed Induction Generator (Average Model)1/Average_VSC/Converter_model ==
  note: P = Vab*Ia -Vbc*Ic = Vdc*Idc
      | Idc = (Vab*Ia -Vbc*Ic)/Vdc
  Ia_Ic : Inport
  Vdc : Inport  Port=2
  Uref : Inport  Port=3
  Add : Sum  Inputs=+-
  Add1 : Sum  Inputs=+-
  Constant : Constant  Value=1e-6
  Delay1 : UnitDelay  SampleTime=Ts  HasFrameUpgradeWarning=on
  Delay2 : UnitDelay  InitialCondition=1e-6  SampleTime=Ts  HasFrameUpgradeWarning=on
  Demux : Demux  Outputs=3
  Demux1 : Demux  Outputs=2
  Gain : Gain  Gain=0.5
  Mult : Product  Inputs=**
  Mux1 : Mux  Inputs=2
  Predictor : Subsystem
  Product3 : Product  RndMeth=Zero
  Product4 : Product  RndMeth=Zero
  Product5 : Product  Inputs=*/  RndMeth=Zero
  Subtract2 : Sum  Inputs=+-
  Subtract3 : Sum
  Idc : Outport
  Vab_Vbc : Outport  Port=2
  wires:
  Mux1/1 -> Vab_Vbc/1
  Uref/1 -> Mult/1
  Vdc/1 -> Delay1/1
  Ia_Ic/1 -> Demux1/1
  Delay2/1 -> Idc/1  "idc"
  Demux1/1 -> Product3/2  "ia"
  Subtract2/1 -> Product5/1  "Pac"
  Product5/1 -> Delay2/1
  Constant/1 -> Subtract3/2
  Subtract3/1 -> Product5/2
  Product4/1 -> Subtract2/2
  Product3/1 -> Subtract2/1
  Demux1/2 -> Product4/2  "ic"
  Add1/1 -> Product4/1, Mux1/2  "Vbc"
  Add/1 -> Product3/1, Mux1/1  "Vab"
  Predictor/1(Out) -> Subtract3/1
  Demux/1 -> Add/1
  Demux/2 -> Add1/1, Add/2
  Demux/3 -> Add1/2
  Mult/1 -> Demux/1
  Gain/1 -> Mult/2
  Delay1/1 -> Predictor/1(In), Gain/1

== system SSN_39busRT_Ctrl_4WT_19B/SM_master/4 WT/SS_windfarm1to2/Wind Farm (DFIG Type)1/Wind Turbine Doubly-Fed Induction Generator (Average Model)1/Average_VSC1/Converter_model ==
  note: P = Vab*Ia -Vbc*Ic = Vdc*Idc
      | Idc = (Vab*Ia -Vbc*Ic)/Vdc
  Ia_Ic : Inport
  Vdc : Inport  Port=2
  Uref : Inport  Port=3
  Add : Sum  Inputs=+-
  Add1 : Sum  Inputs=+-
  Constant : Constant  Value=1e-6
  Delay1 : UnitDelay  SampleTime=Ts  HasFrameUpgradeWarning=on
  Delay2 : UnitDelay  InitialCondition=1e-6  SampleTime=Ts  HasFrameUpgradeWarning=on
  Demux : Demux  Outputs=3
  Demux1 : Demux  Outputs=2
  Gain : Gain  Gain=0.5
  Mult : Product  Inputs=**
  Mux1 : Mux  Inputs=2
  Predictor : Subsystem
  Product3 : Product  RndMeth=Zero
  Product4 : Product  RndMeth=Zero
  Product5 : Product  Inputs=*/  RndMeth=Zero
  Subtract2 : Sum  Inputs=+-
  Subtract3 : Sum
  Idc : Outport
  Vab_Vbc : Outport  Port=2
  wires:
  Mux1/1 -> Vab_Vbc/1
  Uref/1 -> Mult/1
  Vdc/1 -> Delay1/1
  Ia_Ic/1 -> Demux1/1
  Delay2/1 -> Idc/1  "idc"
  Demux1/1 -> Product3/2  "ia"
  Subtract2/1 -> Product5/1  "Pac"
  Product5/1 -> Delay2/1
  Constant/1 -> Subtract3/2
  Subtract3/1 -> Product5/2
  Product4/1 -> Subtract2/2
  Product3/1 -> Subtract2/1
  Demux1/2 -> Product4/2  "ic"
  Add1/1 -> Product4/1, Mux1/2  "Vbc"
  Add/1 -> Product3/1, Mux1/1  "Vab"
  Predictor/1(Out) -> Subtract3/1
  Demux/1 -> Add/1
  Demux/2 -> Add1/1, Add/2
  Demux/3 -> Add1/2
  Mult/1 -> Demux/1
  Gain/1 -> Mult/2
  Delay1/1 -> Predictor/1(In), Gain/1

== system SSN_39busRT_Ctrl_4WT_19B/SM_master/4 WT/SS_windfarm1to2/Wind Farm (DFIG Type)1/Wind Turbine Doubly-Fed Induction Generator (Average Model)1/Control System_average/Control ==
  Vabc_B1 : Inport
  Iabc_grid_conv : Inport  Port=2
  Vdc : Inport  Port=3
  Iabc_stator : Inport  Port=4
  Iabc_rotor : Inport  Port=5
  Q_ref : Inport  Port=6
  Iq_grid_conv_ref : Inport  Port=7
  Q_B1 : Inport  Port=8
  wr : Inport  Port=9
  angle_rotor : Inport  Port=10
  0-pitch_max : Saturate  UpperLimit=pitch_max  LowerLimit=0
  Constant2 : Constant  Value=speed_D
  Discrete 3-phase PLL : powerlib_extras/Discrete  Control Blocks/Discrete 3-phase PLL  Fmin=Fnom-10  Par_Init=[-45 Fnom]  ParK=[60 1400]  Ts=Ts  AGC=off
      settings: SourceProductBaseCode=PS
  Grid-side converter Control system : Subsystem
  Mux : Mux  Inputs=2
  "Rate Limiter   " : RateLimiter  RisingSlewLimit=pitch_rate  FallingSlewLimit=-pitch_rate
  Rotor-side converter Control system : Subsystem
  Sum : Sum  Inputs=|+-  SaturateOnIntegerOverflow=on
  Terminator : Terminator
  pitch_gain : Gain  Gain=pitch_gain  SaturateOnIntegerOverflow=on  OutDataTypeStr=Inherit: Same as input  ParamDataTypeStr=Inherit: Same as input
  Uctrl_grid_conv : Outport
  Uctrl_rotor_conv : Outport  Port=2
  Theta_Freq : Outport  Port=3
  Pitch_angle : Outport  Port=4
  wires:
  Rotor-side converter Control system/1(Uctrl_rotor_conv) -> Uctrl_rotor_conv/1
  Grid-side converter Control system/1(Uctrl_grid_conv) -> Uctrl_grid_conv/1
  [Vdqs] -> Rotor-side converter Control system/11(Vdqs)
  Grid-side converter Control system/2(Vdqs) -> [Vdqs]
  angle_rotor/1 -> Rotor-side converter Control system/9(angle_rotor)
  Q_B1/1 -> Rotor-side converter Control system/8(Q_B1)
  wr/1 -> Rotor-side converter Control system/1(wr), Sum/1
  0-pitch_max/1 -> "Rate Limiter   "/1
  Constant2/1 -> Sum/2
  Sum/1 -> pitch_gain/1
  pitch_gain/1 -> 0-pitch_max/1
  "Rate Limiter   "/1 -> Pitch_angle/1
  Discrete 3-phase PLL/1 -> Rotor-side converter Control system/10(Freq), Mux/2, Grid-side converter Control system/6(Freq)
  Discrete 3-phase PLL/3 -> Terminator/1
  Mux/1 -> Theta_Freq/1
  Discrete 3-phase PLL/2 -> Rotor-side converter Control system/3(Theta), Mux/1, Grid-side converter Control system/3(Theta)
  Q_ref/1 -> Rotor-side converter Control system/7(Q_ref)
  Iabc_rotor/1 -> Rotor-side converter Control system/5(Iabc_rotor)
  Iabc_stator/1 -> Rotor-side converter Control system/4(Iabc_stator)
  Iabc_grid_conv/1 -> Rotor-side converter Control system/6(Iabc_grid_conv), Grid-side converter Control system/2(Iabc_grid_conv)
  Iq_grid_conv_ref/1 -> Grid-side converter Control system/5(Iq_ref)
  Vabc_B1/1 -> Discrete 3-phase PLL/1, Grid-side converter Control system/1(Vabc_B1)
  Vdc/1 -> Rotor-side converter Control system/2(Vdc), Grid-side converter Control system/4(Vdc)

== system SSN_39busRT_Ctrl_4WT_19B/SM_master/4 WT/SS_windfarm1to2/Wind Farm (DFIG Type)1/Wind Turbine Doubly-Fed Induction Generator (Average Model)1/Control System_average/Filter 1000 Hz ==
  Vabc_B1 : Inport
  Iabc_grid_conv : Inport  Port=2
  Vdc : Inport  Port=3
  Iabc_stator : Inport  Port=4
  Iabc_rotor : Inport  Port=5
  Q_ref : Inport  Port=6
  Iq_grid_conv_ref : Inport  Port=7
  Q_B1 : Inport  Port=8
  wr : Inport  Port=9
  angle_rotor : Inport  Port=10
  Demux{,1..3} (4 alike) : Demux  Outputs=3
      settings: DisplayOption=none
  Discrete 2nd-Order Filter{1..14,16..18,20} (18 alike) : powerlib_extras/Discrete  Control Blocks/Discrete  2nd-Order Filter  FilterType=Lowpass  Fo=Freq  Zeta=Zeta  Ts=Ts  Initialize=off  Vac_Init=[0.8 -25 60]  Vdc_Init=-0.4  PlotResponse=off  param1=[1 500 1]
      settings: SourceProductBaseCode=PS
  Mux{,1..3} (4 alike) : Mux  Inputs=3
  "Vabc_B1 " : Outport
  "Iabc_grid_conv " : Outport  Port=2
  "Vdc " : Outport  Port=3
  "Iabc_stator " : Outport  Port=4
  "Iabc_rotor " : Outport  Port=5
  "Q_ref " : Outport  Port=6
  "Iq_grid_conv_ref " : Outport  Port=7
  "Q_B1 " : Outport  Port=8
  "wr " : Outport  Port=9
  "angle_rotor " : Outport  Port=10
  wires:
  Discrete 2nd-Order Filter20/1 -> "Iq_grid_conv_ref "/1
  Iq_grid_conv_ref/1 -> Discrete 2nd-Order Filter20/1
  Mux3/1 -> "Iabc_rotor "/1
  Iabc_rotor/1 -> Demux3/1
  Discrete 2nd-Order Filter16/1 -> Mux3/3
  Discrete 2nd-Order Filter18/1 -> Mux3/2
  Discrete 2nd-Order Filter17/1 -> Mux3/1
  Demux3/3 -> Discrete 2nd-Order Filter16/1
  Demux3/2 -> Discrete 2nd-Order Filter18/1
  Demux3/1 -> Discrete 2nd-Order Filter17/1
  Discrete 2nd-Order Filter11/1 -> "Q_ref "/1
  Discrete 2nd-Order Filter14/1 -> "angle_rotor "/1
  angle_rotor/1 -> Discrete 2nd-Order Filter14/1
  Discrete 2nd-Order Filter13/1 -> "wr "/1
  wr/1 -> Discrete 2nd-Order Filter13/1
  Discrete 2nd-Order Filter12/1 -> "Q_B1 "/1
  Q_B1/1 -> Discrete 2nd-Order Filter12/1
  Q_ref/1 -> Discrete 2nd-Order Filter11/1
  Mux2/1 -> "Iabc_stator "/1
  Iabc_stator/1 -> Demux2/1
  Discrete 2nd-Order Filter10/1 -> Mux2/3
  Discrete 2nd-Order Filter9/1 -> Mux2/2
  Discrete 2nd-Order Filter8/1 -> Mux2/1
  Demux2/3 -> Discrete 2nd-Order Filter10/1
  Demux2/2 -> Discrete 2nd-Order Filter9/1
  Demux2/1 -> Discrete 2nd-Order Filter8/1
  Discrete 2nd-Order Filter7/1 -> "Vdc "/1
  Vdc/1 -> Discrete 2nd-Order Filter7/1
  Mux1/1 -> "Iabc_grid_conv "/1
  Iabc_grid_conv/1 -> Demux1/1
  Discrete 2nd-Order Filter6/1 -> Mux1/3
  Discrete 2nd-Order Filter5/1 -> Mux1/2
  Discrete 2nd-Order Filter4/1 -> Mux1/1
  Demux1/3 -> Discrete 2nd-Order Filter6/1
  Demux1/2 -> Discrete 2nd-Order Filter5/1
  Demux1/1 -> Discrete 2nd-Order Filter4/1
  Mux/1 -> "Vabc_B1 "/1
  Vabc_B1/1 -> Demux/1
  Discrete 2nd-Order Filter3/1 -> Mux/3
  Discrete 2nd-Order Filter2/1 -> Mux/2
  Discrete 2nd-Order Filter1/1 -> Mux/1
  Demux/3 -> Discrete 2nd-Order Filter3/1
  Demux/2 -> Discrete 2nd-Order Filter2/1
  Demux/1 -> Discrete 2nd-Order Filter1/1
